simulink model "sampleModel1435"  (R2023a)
settings: Solver=VariableStepAuto  StartTime=0.0  StopTime=10.0  RelTol=1e-3
libraries: hdlsllib x6, simulink x2
settings Model: Creator=user1  LastModifiedBy=user1

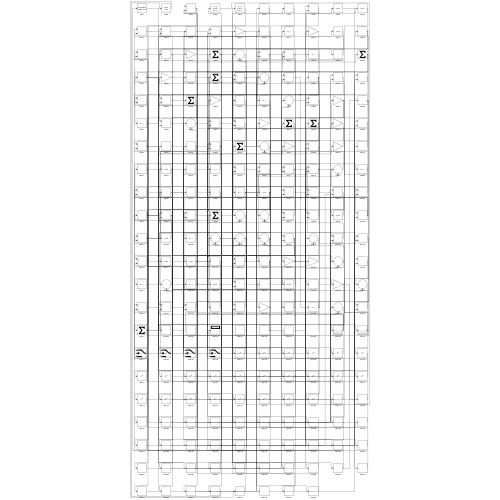
[thumbnail: Simulink's stored preview of the top-level diagram]
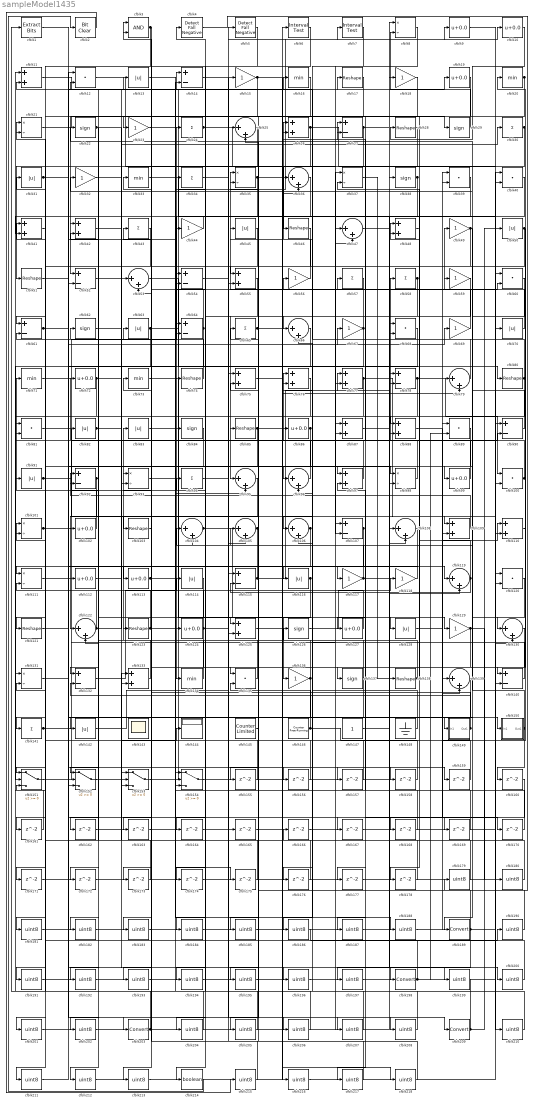
== system sampleModel1435 ==
  cfblk1 : simulink/Logic and Bit Operations/Extract Bits  bitsToExtract=Upper half  numBits=8  bitIdxRange=[0 7]  outScalingMode=Preserve fixed-point scaling
      settings: LibrarySourceBlock=|
      | hdlsllib/Logic and Bit
      | Operations/Extract Bits
  cfblk{9..10,19,72,86,99,102,112..113,124,127} (11 alike) : Bias  Bias=0.0  SaturateOnIntegerOverflow=off
  cfblk{12,39..40,60,68,81,89,100,120,135} (10 alike) : DotProduct  OutDataTypeStr=Inherit: Inherit via internal rule
  cfblk{8,21,35,37,93,98,101,111,131} (9 alike) : Product  Inputs=*/  RndMeth=Zero  SaturateOnIntegerOverflow=on
  cfblk{17,28,46,51,74,80,85,103,121,123,138} (11 alike) : Reshape
  cfblk{25,36,47,53,66,79,95..96,104..106,108,119,122,130,139} (16 alike) : Sum  Inputs=|++
  cfblk{14,27,52,54,61,64,78,90,92,107,115,132,140} (13 alike) : Sum  Inputs=+-
  cfblk{11,26,41..42,48,55,75..77,87..88,97,109..110,125,133} (16 alike) : Sum
  cfblk{13,31,45,50,63,70,82..83,91,114,116,128,142} (13 alike) : Abs  SaturateOnIntegerOverflow=off
  cfblk{15,18,23,32,44,49,56,59,67,69,117..118,129,136} (14 alike) : Gain
  cfblk{22,29,38,62,84,126,137} (7 alike) : Signum
  cfblk{16,20,33,71,73,134} (6 alike) : MinMax
  cfblk{24,30,34,43,57..58,65,94,141} (9 alike) : Sum  Inputs=+
  cfblk143 : Scope
      settings: Floating=on
  cfblk144 : Display
  cfblk145 : hdlsllib/Sources/Counter Limited  uplimit=7  tsamp=-1
  cfblk146 : hdlsllib/Sources/Counter Free-Running  NumBits=16  tsamp=-1
  cfblk147 : Constant  SampleTime=-1
  cfblk148 : Ground
  cfblk149 : Subsystem
      settings: LibrarySourceBlock=|
      | hdlsllib/Ports &
      | Subsystems/Subsystem
  cfblk150 : Subsystem
      settings: LibrarySourceBlock=|
      | hdlsllib/Ports &
      | Subsystems/Subsystem
  cfblk{151..154} (4 alike) : Switch  SaturateOnIntegerOverflow=off  InputSameDT=off
  cfblk{155..178} (24 alike) : Delay  SampleTime=1
  cfblk{179..188,190..197,199..202,204..208,210..213,215..218} (35 alike) : DataTypeConversion  OutDataTypeStr=uint8  SaturateOnIntegerOverflow=off  RndMeth=Floor
  cfblk{189,198,203,209} (4 alike) : DataTypeConversion  SaturateOnIntegerOverflow=off  RndMeth=Floor
  cfblk2 : simulink/Logic and Bit Operations/Bit Clear  iBit=0
      settings: LibrarySourceBlock=|
      | hdlsllib/Logic and Bit
      | Operations/Bit Clear
  cfblk214 : DataTypeConversion  OutDataTypeStr=boolean  SaturateOnIntegerOverflow=off  RndMeth=Floor
  cfblk3 : Logic  AllPortsSameDT=off  OutDataTypeStr=boolean
  cfblk4 : hdlsllib/Logic and Bit Operations/Detect Fall Negative  vinit=0  OutDataTypeStr=boolean
  cfblk5 : hdlsllib/Logic and Bit Operations/Detect Fall Negative  vinit=0  OutDataTypeStr=boolean
  cfblk6 : hdlsllib/Logic and Bit Operations/Interval Test  IntervalClosedRight=on  uplimit=0.5  IntervalClosedLeft=on  lowlimit=-0.5  OutDataTypeStr=boolean
  cfblk7 : hdlsllib/Logic and Bit Operations/Interval Test  IntervalClosedRight=on  uplimit=0.5  IntervalClosedLeft=on  lowlimit=-0.5  OutDataTypeStr=boolean
  wires:
  cfblk67/1 -> cfblk66/1, cfblk154/3
  cfblk37/1 -> cfblk138/1
  cfblk153/1 -> cfblk17/1
  cfblk85/1 -> cfblk77/1, cfblk152/3, cfblk27/1, cfblk218/1
  cfblk55/1 -> cfblk95/1
  cfblk98/1 -> cfblk58/1
  cfblk73/1 -> cfblk128/1
  cfblk53/1 -> cfblk80/1
  cfblk7/1 -> cfblk77/2
  cfblk30/1 -> cfblk51/1, cfblk193/1
  cfblk106/1 -> cfblk201/1, cfblk213/1
  cfblk140/1 -> cfblk66/2
  cfblk104/1 -> cfblk129/1, cfblk57/1
  cfblk84/1 -> cfblk151/1
  cfblk115/1 -> cfblk78/1, cfblk113/1
  cfblk21/1 -> cfblk29/1
  cfblk68/1 -> cfblk97/1
  cfblk17/1 -> cfblk52/1
  cfblk137/1 -> cfblk62/1, cfblk111/2, cfblk152/2
  cfblk35/1 -> cfblk134/1, cfblk79/2
  cfblk141/1 -> cfblk24/1, cfblk16/1
  cfblk44/1 -> cfblk42/1
  cfblk102/1 -> cfblk71/1
  cfblk150/1(Out1) -> cfblk32/1, cfblk104/1, cfblk160/1
  cfblk69/1 -> cfblk35/1
  cfblk79/1 -> cfblk45/1
  cfblk94/1 -> cfblk7/1
  cfblk63/1 -> cfblk9/1, cfblk93/2
  cfblk92/1 -> cfblk122/1, cfblk12/2
  cfblk146/1 -> cfblk20/1, cfblk65/1
  cfblk16/1 -> cfblk55/1
  cfblk126/1 -> cfblk118/1
  cfblk118/1 -> cfblk117/1
  cfblk56/1 -> cfblk26/1
  cfblk10/1 -> cfblk28/1
  cfblk135/1 -> cfblk83/1
  cfblk116/1 -> cfblk136/1, cfblk194/1
  cfblk100/1 -> cfblk76/1, cfblk73/1, cfblk27/2
  cfblk97/1 -> cfblk33/1
  cfblk111/1 -> cfblk69/1
  cfblk28/1 -> cfblk52/2
  cfblk71/1 -> cfblk63/1
  cfblk86/1 -> cfblk132/1, cfblk161/1
  cfblk81/1 -> cfblk109/1
  cfblk131/1 -> cfblk203/1
  cfblk12/1 -> cfblk46/1
  cfblk132/1 -> cfblk114/1
  cfblk8/1 -> cfblk106/1
  cfblk123/1 -> cfblk41/1, cfblk88/2, cfblk188/1
  cfblk25/1 -> cfblk55/2
  cfblk151/1 -> cfblk47/1
  cfblk15/1 -> cfblk141/1, cfblk167/1
  cfblk26/1 -> cfblk85/1, cfblk90/1
  cfblk62/1 -> cfblk119/1
  cfblk20/1 -> cfblk103/1, cfblk88/1
  cfblk101/1 -> cfblk12/1, cfblk14/2, cfblk207/1
  cfblk138/1 -> cfblk76/2, cfblk48/1
  cfblk23/1 -> cfblk84/1
  cfblk128/1 -> cfblk110/1
  cfblk74/1 -> cfblk21/1
  cfblk110/1 -> cfblk130/1
  cfblk43/1 -> cfblk142/1
  cfblk103/1 -> cfblk3/1
  cfblk77/1 -> cfblk130/2, cfblk135/1
  cfblk59/1 -> cfblk106/2
  cfblk124/1 -> cfblk15/1, cfblk21/2, cfblk173/1, cfblk174/1
  cfblk13/1 -> cfblk154/1
  cfblk99/1 -> cfblk72/1
  cfblk9/1 -> cfblk110/2
  cfblk113/1 -> cfblk95/2, cfblk56/1
  cfblk34/1 -> cfblk209/1
  cfblk11/1 -> cfblk19/1
  cfblk65/1 -> cfblk60/2, cfblk59/1
  cfblk127/1 -> cfblk42/2
  cfblk24/1 -> cfblk107/1, cfblk214/1
  cfblk49/1 -> cfblk149/1(In1), cfblk177/1, cfblk185/1
  cfblk27/1 -> cfblk10/1, cfblk125/2
  cfblk107/1 -> cfblk125/1, cfblk171/1, cfblk172/1
  cfblk125/1 -> cfblk6/1
  cfblk129/1 -> cfblk163/1, cfblk180/1
  cfblk142/1 -> cfblk25/1
  cfblk46/1 -> cfblk61/1
  cfblk136/1 -> cfblk94/1, cfblk212/1
  cfblk122/1 -> cfblk53/1, cfblk101/1
  cfblk76/1 -> cfblk111/1
  cfblk64/1 -> cfblk151/2, cfblk3/2
  cfblk90/1 -> cfblk22/1
  cfblk41/1 -> cfblk121/1
  cfblk119/1 -> cfblk115/2, cfblk37/2
  cfblk50/1 -> cfblk140/1, cfblk153/2
  cfblk149/1(Out1) -> cfblk53/2, cfblk93/1, cfblk132/2
  cfblk51/1 -> cfblk44/1
  cfblk147/1 -> cfblk8/1
  cfblk148/1 -> cfblk126/1
  cfblk29/1 -> cfblk8/2
  cfblk47/1 -> cfblk18/1
  cfblk133/1 -> cfblk81/1
  cfblk31/1 -> cfblk116/1, cfblk74/1, cfblk168/1
  cfblk42/1 -> cfblk14/1
  cfblk154/1 -> cfblk68/1
  cfblk112/1 -> cfblk153/1
  cfblk61/1 -> cfblk150/1(In1), cfblk159/1
  cfblk38/1 -> cfblk96/1, cfblk41/2, cfblk98/2
  cfblk72/1 -> cfblk101/2, cfblk158/1
  cfblk58/1 -> cfblk96/2, cfblk127/1
  cfblk3/1 -> cfblk23/1, cfblk191/1
  cfblk19/1 -> cfblk26/2
  cfblk134/1 -> cfblk82/1
  cfblk66/1 -> cfblk124/1
  cfblk22/1 -> cfblk107/2, cfblk102/1
  cfblk117/1 -> cfblk119/2, cfblk90/2, cfblk104/2
  cfblk152/1 -> cfblk144/1
  cfblk82/1 -> cfblk133/2, cfblk30/1
  cfblk70/1 -> cfblk49/1
  cfblk96/1 -> cfblk31/1
  cfblk1/1 -> cfblk198/1
  cfblk120/1 -> cfblk189/1
  cfblk60/1 -> cfblk99/1
  cfblk91/1 -> cfblk64/2, cfblk98/1, cfblk67/1
  cfblk109/1 -> cfblk92/1
  cfblk78/1 -> cfblk152/1, cfblk100/1
  cfblk105/1 -> cfblk153/3, cfblk155/1
  cfblk18/1 -> cfblk137/1
  cfblk80/1 -> cfblk11/2, cfblk176/1
  cfblk145/1 -> cfblk25/2
  cfblk155/1 -> cfblk92/2
  cfblk52/1 -> cfblk156/1
  cfblk156/1 -> cfblk35/2
  cfblk83/1 -> cfblk157/1
  cfblk157/1 -> cfblk64/1
  cfblk158/1 -> cfblk81/2
  cfblk159/1 -> cfblk89/1
  cfblk161/1 -> cfblk11/1
  cfblk114/1 -> cfblk162/1
  cfblk162/1 -> cfblk78/2
  cfblk163/1 -> cfblk100/2
  cfblk57/1 -> cfblk164/1
  cfblk164/1 -> cfblk109/2
  cfblk14/1 -> cfblk165/1
  cfblk166/1 -> cfblk47/2
  cfblk168/1 -> cfblk97/2
  cfblk121/1 -> cfblk169/1
  cfblk169/1 -> cfblk154/2
  cfblk88/1 -> cfblk170/1
  cfblk170/1 -> cfblk115/1
  cfblk171/1 -> cfblk68/2
  cfblk172/1 -> cfblk140/2
  cfblk173/1 -> cfblk122/2
  cfblk93/1 -> cfblk175/1
  cfblk175/1 -> cfblk133/1
  cfblk176/1 -> cfblk151/3
  cfblk177/1 -> cfblk79/1
  cfblk48/1 -> cfblk178/1
  cfblk178/1 -> cfblk37/1
  cfblk4/1 -> cfblk179/1
  cfblk179/1 -> cfblk86/1
  cfblk180/1 -> cfblk4/1
  cfblk5/1 -> cfblk181/1
  cfblk181/1 -> cfblk70/1
  cfblk45/1 -> cfblk182/1
  cfblk182/1 -> cfblk5/1
  cfblk39/1 -> cfblk183/1
  cfblk183/1 -> cfblk38/1
  cfblk6/1 -> cfblk184/1
  cfblk184/1 -> cfblk39/1
  cfblk185/1 -> cfblk39/2
  cfblk139/1 -> cfblk186/1
  cfblk130/1 -> cfblk187/1
  cfblk187/1 -> cfblk139/1
  cfblk188/1 -> cfblk139/2
  cfblk189/1 -> cfblk135/2, cfblk197/1
  cfblk186/1 -> cfblk190/1
  cfblk190/1 -> cfblk120/1
  cfblk191/1 -> cfblk120/2
  cfblk40/1 -> cfblk192/1
  cfblk192/1 -> cfblk105/2
  cfblk193/1 -> cfblk40/1
  cfblk194/1 -> cfblk40/2
  cfblk108/1 -> cfblk195/1
  cfblk195/1 -> cfblk105/1
  cfblk32/1 -> cfblk196/1
  cfblk196/1 -> cfblk108/1
  cfblk197/1 -> cfblk108/2
  cfblk198/1 -> cfblk61/2, cfblk89/2
  cfblk167/1 -> cfblk199/1
  cfblk199/1 -> cfblk1/1
  cfblk87/1 -> cfblk200/1
  cfblk200/1 -> cfblk123/1
  cfblk201/1 -> cfblk87/1
  cfblk95/1 -> cfblk202/1
  cfblk202/1 -> cfblk87/2
  cfblk203/1 -> cfblk48/2, cfblk91/1
  cfblk89/1 -> cfblk204/1
  cfblk204/1 -> cfblk131/1
  cfblk165/1 -> cfblk205/1
  cfblk205/1 -> cfblk131/2
  cfblk54/1 -> cfblk206/1
  cfblk206/1 -> cfblk13/1
  cfblk207/1 -> cfblk54/1
  cfblk174/1 -> cfblk208/1
  cfblk208/1 -> cfblk54/2
  cfblk209/1 -> cfblk166/1, cfblk50/1
  cfblk33/1 -> cfblk210/1
  cfblk210/1 -> cfblk34/1
  cfblk36/1 -> cfblk211/1
  cfblk211/1 -> cfblk112/1
  cfblk212/1 -> cfblk36/1
  cfblk213/1 -> cfblk36/2
  cfblk214/1 -> cfblk2/1
  cfblk2/1 -> cfblk215/1
  cfblk215/1 -> cfblk43/1
  cfblk75/1 -> cfblk216/1
  cfblk216/1 -> cfblk60/1
  cfblk160/1 -> cfblk217/1
  cfblk217/1 -> cfblk75/1
  cfblk218/1 -> cfblk75/2

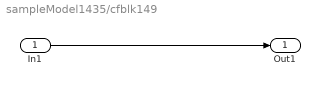
== system sampleModel1435/cfblk149 ==
  In1 : Inport
  Out1 : Outport
  wires:
  In1/1 -> Out1/1

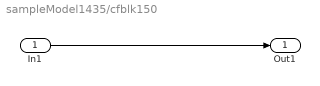
== system sampleModel1435/cfblk150 ==
  In1 : Inport
  Out1 : Outport
  wires:
  In1/1 -> Out1/1
